simulink model "ObserverDesignControl_sol"  (R2024b)
settings: Solver=VariableStepAuto  StartTime=0.0  StopTime=10.0  RelTol=1e-3
settings Model: Creator=auw_a  LastModifiedBy=auw_a

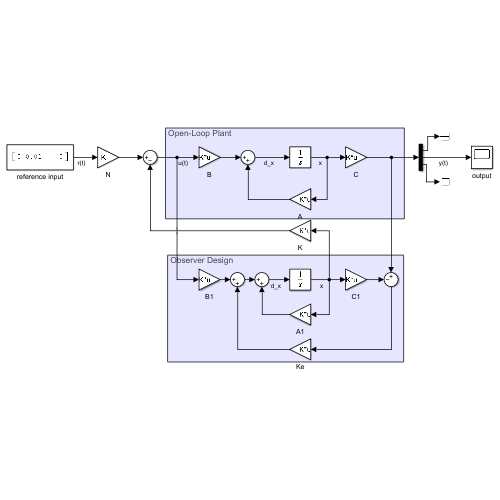
[thumbnail: Simulink's stored preview of the top-level diagram]
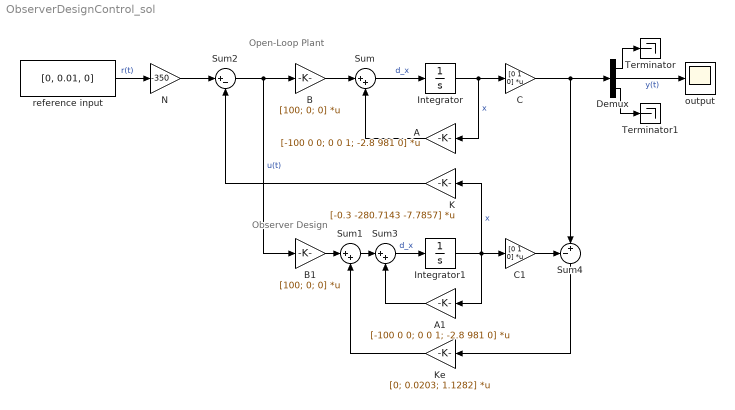
== system ObserverDesignControl_sol ==
  note: Observer Design
  note: Open-Loop Plant
  A : Gain  Gain=[-100 0 0; 0 0 1; -2.8 981 0]  Multiplication=Matrix(K*u)
  A1 : Gain  Gain=[-100 0 0; 0 0 1; -2.8 981 0]  Multiplication=Matrix(K*u)
  B : Gain  Gain=[100; 0; 0]  Multiplication=Matrix(K*u)
  B1 : Gain  Gain=[100; 0; 0]  Multiplication=Matrix(K*u)
  C : Gain  Gain=[0 1 0]  Multiplication=Matrix(K*u)
  C1 : Gain  Gain=[0 1 0]  Multiplication=Matrix(K*u)
  Demux : Demux  Outputs=3
  Integrator : Integrator
  Integrator1 : Integrator
  K : Gain  Gain=[-0.3 -280.7143 -7.7857]  Multiplication=Matrix(K*u)
  Ke : Gain  Gain=[0; 0.0203; 1.1282]  Multiplication=Matrix(K*u)
  N : Gain  Gain=-350
  Sum : Sum  Inputs=|++
  Sum1 : Sum  Inputs=|++
  Sum2 : Sum  Inputs=|+-
  Sum3 : Sum  Inputs=|++
  Sum4 : Sum  Inputs=-+|
  Terminator : Terminator
  Terminator1 : Terminator
  output : Scope
  reference input : Constant  Value=[0, 0.01, 0]  VectorParams1D=off
  wires:
  B/1 -> Sum/1
  A/1 -> Sum/2
  Sum/1 -> Integrator/1  "d_x"
  Integrator/1 -> A/1, C/1  "x"
  Sum2/1 -> B/1, B1/1  "u(t)"
  reference input/1 -> N/1  "r(t)"
  K/1 -> Sum2/2
  C/1 -> Demux/1, Sum4/2
  Demux/1 -> Terminator/1
  Demux/2 -> output/1  "y(t)"
  Demux/3 -> Terminator1/1
  N/1 -> Sum2/1
  Ke/1 -> Sum1/2
  Integrator1/1 -> C1/1, A1/1, K/1  "x"
  Sum3/1 -> Integrator1/1  "d_x"
  A1/1 -> Sum3/2
  Sum4/1 -> Ke/1
  C1/1 -> Sum4/1
  B1/1 -> Sum1/1
  Sum1/1 -> Sum3/1
